simulink model "test_kinematic_model"  (R2019b)
settings: Solver=VariableStepAuto  StartTime=0.0  StopTime=10  RelTol=1e-3
libraries: simulink x2
settings Model: Creator=jiyo  LastModifiedBy=jiyo

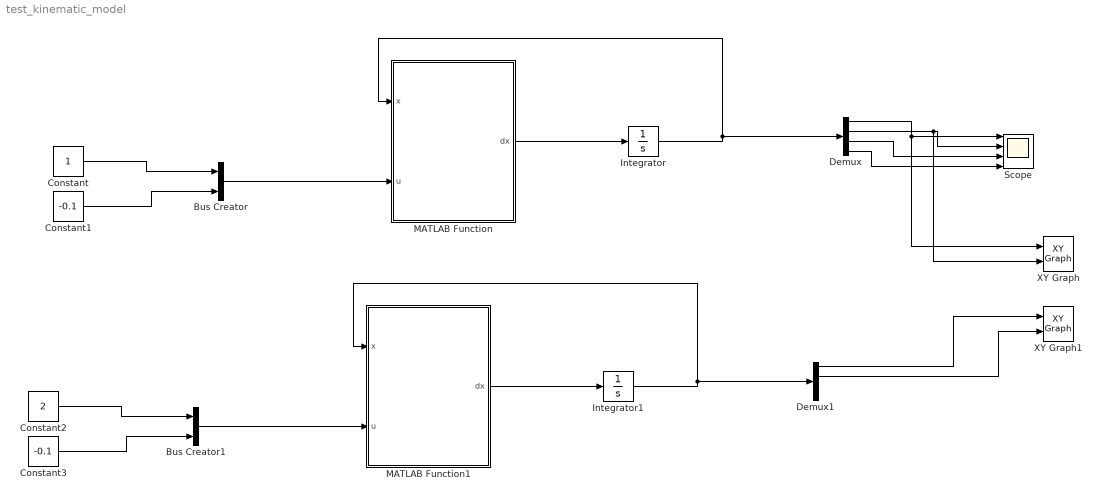
== system test_kinematic_model ==
  Bus Creator : BusCreator  Inputs=2
  Bus Creator1 : BusCreator  Inputs=2
  Constant : Constant  OutDataTypeStr=double
  Constant1 : Constant  Value=-0.1  OutDataTypeStr=double
  Constant2 : Constant  Value=2  OutDataTypeStr=double
  Constant3 : Constant  Value=-0.1  OutDataTypeStr=double
  Demux : Demux
  Demux1 : Demux
  Integrator : Integrator  InitialCondition=[0.0 0.0 0.0 0.0]
  Integrator1 : Integrator  InitialCondition=[0.0 0.0 0.0 0.0]
  MATLAB Function : MATLAB Function  TreatAsAtomicUnit=on
  MATLAB Function1 : MATLAB Function  TreatAsAtomicUnit=on
  Scope : Scope  NumInputPorts=4
  XY Graph : simulink/Sinks/XY Graph  xmin=-30  xmax=30  ymin=-30  ymax=30  st=-1
  XY Graph1 : simulink/Sinks/XY Graph  xmin=-30  xmax=30  ymin=-30  ymax=30  st=-1
  wires:
  MATLAB Function/1(dx) -> Integrator/1
  Integrator/1 -> Demux/1, MATLAB Function/1(x)
  Bus Creator/1 -> MATLAB Function/2(u)
  Constant/1 -> Bus Creator/1
  Constant1/1 -> Bus Creator/2
  Demux/1 -> XY Graph/1, Scope/1
  Demux/2 -> XY Graph/2, Scope/2
  Demux/3 -> Scope/3
  Demux/4 -> Scope/4
  Constant3/1 -> Bus Creator1/2
  Constant2/1 -> Bus Creator1/1
  Bus Creator1/1 -> MATLAB Function1/2(u)
  Integrator1/1 -> Demux1/1, MATLAB Function1/1(x)
  MATLAB Function1/1(dx) -> Integrator1/1
  Demux1/1 -> XY Graph1/1
  Demux1/2 -> XY Graph1/2

== matlab function test_kinematic_model/MATLAB Function1 ==
  data: x input; u input; dx output
function dx = fcn(x,u)
dx = vkinematicmodel_bicycle(x,u);

== matlab function test_kinematic_model/MATLAB Function ==
  data: x input; u input; dx output
function dx = fcn(x,u)
dx = vkinematicmodel_bicycle(x,u);
